simulink model "ORMComponent_1"  (R2024a)
settings: Solver=FixedStepAuto  StartTime=0.0  StopTime=10.0  RelTol=1e-3
undefined symbols (not defined in the file or in its folder): Client
settings Model: DataDictionary=untitled_dict1.sldd  Creator=diell  LastModifiedBy=diell
settings OptimizationCC: DefaultParameterBehavior=Inlined  OptimizeBlockIOStorage=off  EnhancedBackFolding=on  PassReuseOutputArgsThreshold=0  OptimizeDataStoreBuffers=off  BusAssignmentInplaceUpdate=off
settings DebuggingCC: ParameterTunabilityLossMsg=error  SFUnexpectedBacktrackingDiag=warning  SFNoUnconditionalDefaultTransitionDiag=warning
settings SFSimCC: MATLABDynamicMemAlloc=off
settings RTWCC: GenerateReport=on  BuildConfiguration=Debug  LaunchReport=on
settings CodeAppCC: ForceParamTrailComments=on  OperatorAnnotations=on  MATLABSourceComments=on  EnableCustomComments=on
settings GRTTargetCC: CombineSignalStateStructs=on  SupportVariableSizeSignals=on  MultiInstanceErrorCode=Warning

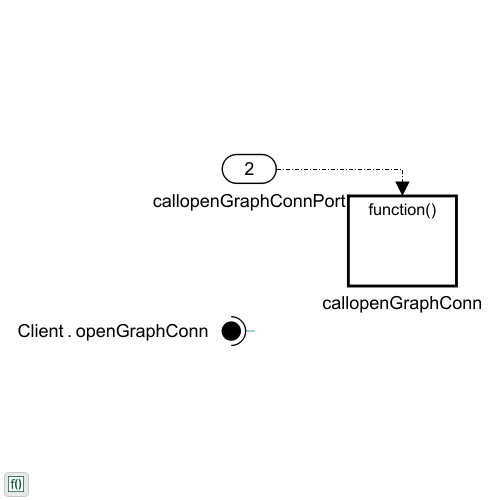
[thumbnail: Simulink's stored preview of the top-level diagram]
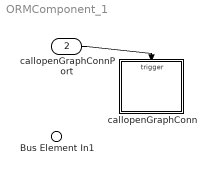
== system ORMComponent_1 ==
  Bus Element In1 : Inport  AllowServiceAccess=on  PortName=Client  Element=openGraphConn
  callopenGraphConnPort : Inport  Port=2  OutputFunctionCall=on
  callopenGraphConn : Subsystem
  wires:
  callopenGraphConnPort/1 -> callopenGraphConn/Trigger

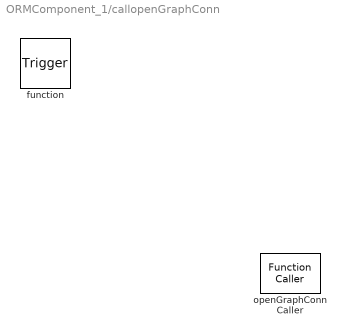
== system ORMComponent_1/callopenGraphConn ==
  function : TriggerPort  TriggerType=function-call  VariantControl=(inherit)
  openGraphConn Caller : FunctionCaller  FunctionPrototype=Client.openGraphConn()  InputArgumentSpecifications=<Enter example>  OutputArgumentSpecifications=<Enter example>
